simulink model "DimmerCircuit_fromzero_tomax"  (R2024a)
settings: Solver=VariableStepAuto  StartTime=0.0  StopTime=inf  RelTol=1e-3
libraries: arduinolib x1
settings Model: Creator=VICTUS  LastModifiedBy=VICTUS

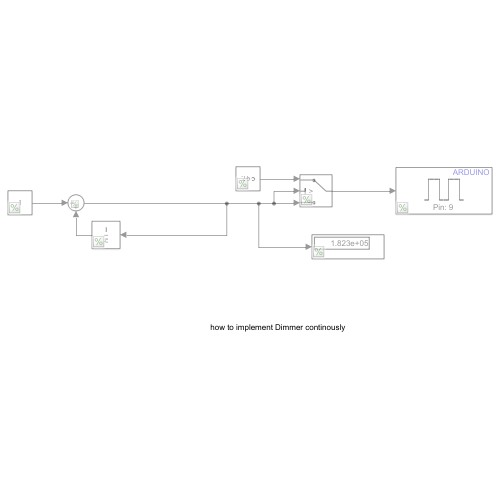
[thumbnail: Simulink's stored preview of the top-level diagram]
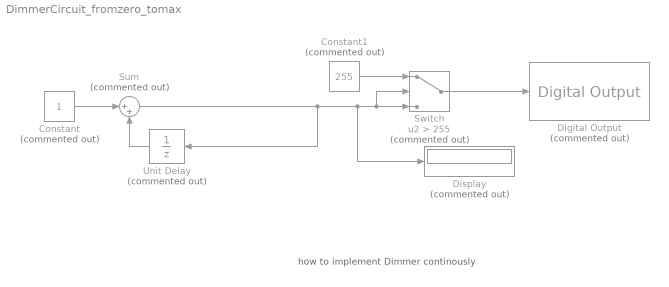
== system DimmerCircuit_fromzero_tomax ==
  note: how to implement Dimmer continously
  Constant : Constant  Commented=on
  Constant1 : Constant  Commented=on  Value=255
  Digital Output : arduinolib/Digital Output  Commented=on  pinNumber=9  Direction=output  blockPlatform=arduino
  Display : Display  Commented=on
  Sum : Sum  Commented=on  Inputs=|++
  Switch : Switch  Commented=on  Criteria=u2 > Threshold  Threshold=255  SaturateOnIntegerOverflow=off  InputSameDT=off
  Unit Delay : UnitDelay  Commented=on  SampleTime=0.003  HasFrameUpgradeWarning=on
  wires:
  Constant/1 -> Sum/1
  Sum/1 -> Unit Delay/1, Display/1, Switch/2, Switch/3
  Unit Delay/1 -> Sum/2
  Switch/1 -> Digital Output/1
  Constant1/1 -> Switch/1
